simulink model "mconversionBusLabel"  (Simulink 8.0)
settings: Solver=FixedStepDiscrete  StartTime=0.0  StopTime=10.0  RelTol=1e-3
settings Model: Creator=awarlock  LastModifiedBy=htu  ExtModeAutoUpdateStatusClock=off
settings DataIOCC: SignalLoggingSaveFormat=ModelDataLogs
settings OptimizationCC: InlineParams=on  InlineInvariantSignals=on  InitFltsAndDblsToZero=on
settings DebuggingCC: SaveWithParameterizedLinksMsg=none  SignalResolutionControl=TryResolveAllWithWarning  MultiTaskDSMMsg=warning  MultiTaskCondExecSysMsg=none
settings SFSimCC: SimParseCustomCode=off
settings RTWCC: IncludeERTFirstTime=on
settings GRTTargetCC: TargetFcnLib=ansi_tfl_tmw.mat  CombineOutputUpdateFcns=off  GRTInterface=on

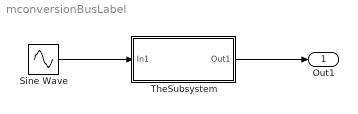
== system mconversionBusLabel ==
  Sine Wave : Sin  SampleTime=0.1
  TheSubsystem : Subsystem  TreatAsAtomicUnit=on
  Out1 : Outport
  wires:
  Sine Wave/1 -> TheSubsystem/1(In1)
  TheSubsystem/1(Out1) -> Out1/1

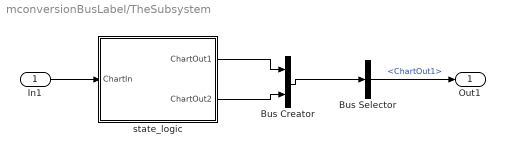
== system mconversionBusLabel/TheSubsystem ==
  In1 : Inport
  Bus Creator : BusCreator  DialogController=Simulink.DDGSource_Bus  Inputs=2
  Bus Selector : BusSelector  DialogController=Simulink.DDGSource_Bus  OutputSignals=ChartOut1
  state_logic : Stateflow chart  TreatAsAtomicUnit=on
  Out1 : Outport
  wires:
  Bus Creator/1 -> Bus Selector/1
  Bus Selector/1 -> Out1/1  "<ChartOut1>"
  state_logic/1(ChartOut1) -> Bus Creator/1
  state_logic/2(ChartOut2) -> Bus Creator/2
  In1/1 -> state_logic/1(ChartIn)

== stateflow chart TheSubsystem/state_logic ==
  settings: updateMethod=DISCRETE  sampleTime=0.1
  state state_of_motion
    state stuck/
      entry:ChartOut1 = 1;
      ChartOut2 = -2;
    state sliding/
      entry: ChartOut1 = 0;
    state blah/
      entry: ChartOut2 = -1
    stuck -> sliding : [ChartIn > 0.3]
    (default) -> stuck
    blah -> stuck : [ChartIn<-0.3]
    sliding -> blah : [(ChartIn)<= 0]
  data: ChartOut1 output double [0..1]; ChartIn input double; ChartOut2 output double
